simulink model "SNL_S_Function"  (R2020b)
settings: Solver=VariableStepAuto  StartTime=0.0  StopTime=10.0  RelTol=1e-3
settings Model: Creator=ashahn  LastModifiedBy=ashahn

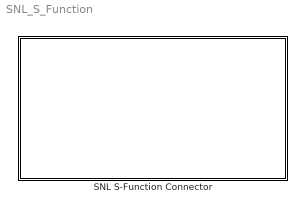
== system SNL_S_Function ==
  SNL S-Function Connector : Subsystem

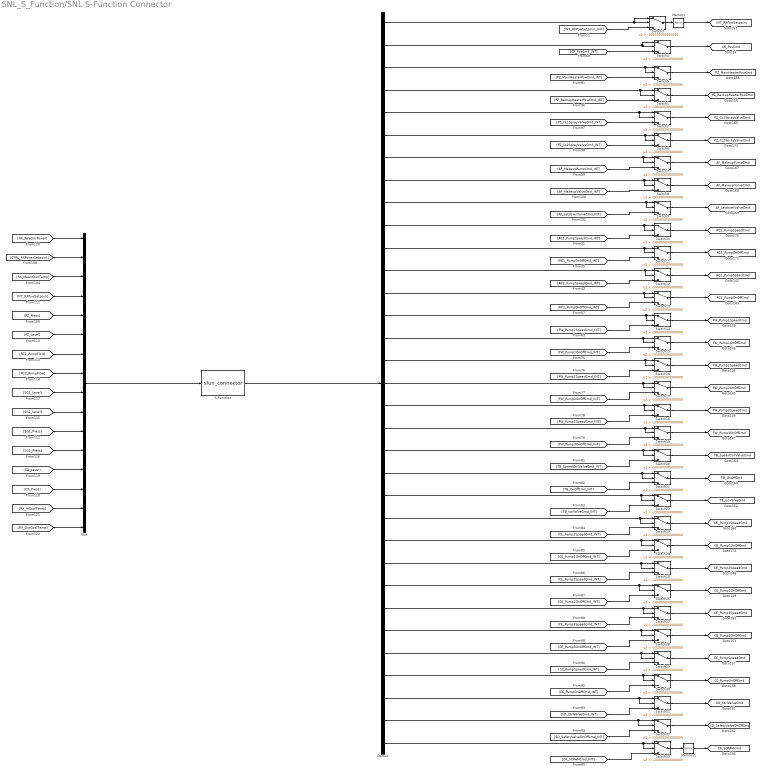
== system SNL_S_Function/SNL S-Function Connector ==
  Demux : Demux  Outputs=33
  Memory : Memory
  Memory1 : Memory
  Mux : Mux  Inputs=16
  S-Function : S-Function  FunctionName=sfun_connector  Parameters='RX_ReactorPower;CTRL_RXPowerSetpoint;RX_MeanCoolTemp;INT_RXPowSetpoint;PZ_Press;PZ_Level;RC1_PumpFlow;RC2_PumpFlow;SG1_Level;SG2_Level;SG1_Press;SG2_Press;CD_Level;CD_Press;RX_InCoolTemp;RX_OutCoolTemp','INT_RXPowSetpoint;CR_PosCmd;PZ_MainHeaterPowCmd;PZ_BackupHeaterPowCmd;PZ_CL1SprayValveCmd;PZ_CL2SprayValveCmd;AF_MakeupPumpCmd;AF_MakeupValveCmd;AF_LetdownValveCmd;RC1_PumpSpeedCmd;RC1_PumpOnOffCmd;RC2_PumpSpeedCmd;RC2_PumpOnOffCmd;FW_Pump1SpeedCmd;FW_Pump1OnOffCmd;FW_Pump2SpeedCmd;FW_Pump2OnOffCmd;FW_Pump3SpeedCmd;FW_Pump3OnOffCmd;TB_SpeedCtrlValveCmd;TB_OnOffCmd;TB_IsoValveCmd;CE_Pump1SpeedCmd;CE_Pump1OnOffCmd;CE_Pump2SpeedCmd;CE_Pump2OnOffCmd;CE_Pump3SpeedCmd;CE_Pump3OnOffCmd;CC_PumpSpeedCmd;CC_PumpOnOffCmd;SD_CtrlValveCmd;SD_SafetyValveOnOffCmd;CR_SCRAMCmd'  SFunctionDeploymentMode=off  EnableBusSupport=off
  Switch{1..33} (33 alike) : Switch  Criteria=u2 > Threshold  Threshold=-100000000000000
  tag scope: AF_LetdownValveCmd=global, AF_MakeupPumpCmd=global, AF_MakeupValveCmd=global, CC_PumpOnOffCmd=global, CC_PumpSpeedCmd=global, CE_Pump1OnOffCmd=global, CE_Pump1SpeedCmd=global, CE_Pump2OnOffCmd=global, CE_Pump2SpeedCmd=global, CE_Pump3OnOffCmd=global, CE_Pump3SpeedCmd=global, CR_PosCmd=global, CR_SCRAMCmd=global, FW_Pump1OnOffCmd=global, FW_Pump1SpeedCmd=global, FW_Pump2OnOffCmd=global, FW_Pump2SpeedCmd=global, FW_Pump3OnOffCmd=global, FW_Pump3SpeedCmd=global, INT_RXPowSetpoint=global, PZ_BackupHeaterPowCmd=global, PZ_CL1SprayValveCmd=global, PZ_CL2SprayValveCmd=global, PZ_MainHeaterPowCmd=global, RC1_PumpOnOffCmd=global, RC1_PumpSpeedCmd=global, RC2_PumpOnOffCmd=global, RC2_PumpSpeedCmd=global, SD_CtrlValveCmd=global, SD_SafetyValveOnOffCmd=global, TB_IsoValveCmd=global, TB_OnOffCmd=global, TB_SpeedCtrlValveCmd=global
  wires:
  [PZ_Level] -> Mux/6
  Demux/29 -> Switch29/2, Switch29/1
  Switch24/1 -> [CE_Pump1OnOffCmd]
  [PZ_CL1SprayValveCmd_INT] -> Switch2/3
  Switch13/1 -> [RC2_PumpOnOffCmd]
  Switch28/1 -> [CE_Pump3OnOffCmd]
  Switch19/1 -> [FW_Pump3OnOffCmd]
  Demux/6 -> Switch6/2, Switch6/1
  Switch12/1 -> [RC2_PumpSpeedCmd]
  [FW_Pump2OnOffCmd_INT] -> Switch17/3
  Demux/22 -> Switch22/2, Switch22/1
  Demux/13 -> Switch13/2, Switch13/1
  [FW_Pump1OnOffCmd_INT] -> Switch15/3
  Demux/30 -> Switch30/2, Switch30/1
  [RX_ReactorPower] -> Mux/1
  Demux/8 -> Switch8/2, Switch8/1
  Switch29/1 -> [CC_PumpSpeedCmd]
  [CE_Pump1SpeedCmd_INT] -> Switch23/3
  Switch14/1 -> [FW_Pump1SpeedCmd]
  Switch26/1 -> [CE_Pump2OnOffCmd]
  [TB_SpeedCtrlValveCmd_INT] -> Switch20/3
  [RX_MeanCoolTemp] -> Mux/3
  Demux/32 -> Switch32/2, Switch32/1
  [CC_PumpOnOffCmd_INT] -> Switch30/3
  Switch1/1 -> [PZ_BackupHeaterPowCmd]
  [CTRL_RXPowerSetpoint] -> Mux/2
  [SG2_Level] -> Mux/10
  [CE_Pump3SpeedCmd_INT] -> Switch27/3
  [SG1_Level] -> Mux/9
  Demux/16 -> Switch16/2, Switch16/1
  Switch6/1 -> [PZ_CL2SprayValveCmd]
  Switch17/1 -> [FW_Pump2OnOffCmd]
  [CE_Pump1OnOffCmd_INT] -> Switch24/3
  [FW_Pump3OnOffCmd_INT] -> Switch19/3
  [PZ_MainHeaterPowCmd_INT] -> Switch5/3
  Switch16/1 -> [FW_Pump2SpeedCmd]
  [FW_Pump2SpeedCmd_INT] -> Switch16/3
  [CE_Pump3OnOffCmd_INT] -> Switch28/3
  Switch25/1 -> [CE_Pump2SpeedCmd]
  Switch7/1 -> [AF_MakeupPumpCmd]
  Demux/19 -> Switch19/2, Switch19/1
  Demux/15 -> Switch15/2, Switch15/1
  [SD_SafetyValveOnOffCmd_INT] -> Switch32/3
  [CE_Pump2SpeedCmd_INT] -> Switch25/3
  Demux/12 -> Switch12/2, Switch12/1
  Demux/17 -> Switch17/2, Switch17/1
  Switch9/1 -> [AF_LetdownValveCmd]
  Switch22/1 -> [TB_IsoValveCmd]
  Switch30/1 -> [CC_PumpOnOffCmd]
  [RX_OutCoolTemp] -> Mux/16
  Demux/25 -> Switch25/2, Switch25/1
  Switch4/1 -> [CR_PosCmd]
  [AF_LetdownValveCmd_INT] -> Switch9/3
  [RC1_PumpSpeedCmd_INT] -> Switch10/3
  [RC2_PumpSpeedCmd_INT] -> Switch12/3
  Demux/3 -> Switch5/2, Switch5/1
  Demux/31 -> Switch31/2, Switch31/1
  [RC2_PumpOnOffCmd_INT] -> Switch13/3
  [TB_IsoValveCmd_INT] -> Switch22/3
  Demux/9 -> Switch9/2, Switch9/1
  [CD_Level] -> Mux/13
  [TB_OnOffCmd_INT] -> Switch21/3
  Switch2/1 -> [PZ_CL1SprayValveCmd]
  Demux/4 -> Switch1/2, Switch1/1
  Demux/26 -> Switch26/2, Switch26/1
  Switch15/1 -> [FW_Pump1OnOffCmd]
  [CC_PumpSpeedCmd_INT] -> Switch29/3
  Switch8/1 -> [AF_MakeupValveCmd]
  Switch23/1 -> [CE_Pump1SpeedCmd]
  [CD_Press] -> Mux/14
  Switch20/1 -> [TB_SpeedCtrlValveCmd]
  Switch10/1 -> [RC1_PumpSpeedCmd]
  Demux/2 -> Switch4/1, Switch4/2
  Demux/28 -> Switch28/2, Switch28/1
  [FW_Pump1SpeedCmd_INT] -> Switch14/3
  Switch31/1 -> [SD_CtrlValveCmd]
  Mux/1 -> S-Function/1
  Switch21/1 -> [TB_OnOffCmd]
  [SG2_Press] -> Mux/12
  [RC2_PumpFlow] -> Mux/8
  [SD_CtrlValveCmd_INT] -> Switch31/3
  Demux/5 -> Switch2/2, Switch2/1
  Demux/21 -> Switch21/2, Switch21/1
  Demux/27 -> Switch27/2, Switch27/1
  [AF_MakeupValveCmd_INT] -> Switch8/3
  Switch11/1 -> [RC1_PumpOnOffCmd]
  Demux/10 -> Switch10/2, Switch10/1
  [FW_Pump3SpeedCmd_INT] -> Switch18/3
  Switch27/1 -> [CE_Pump3SpeedCmd]
  [RC1_PumpFlow] -> Mux/7
  Demux/1 -> Switch3/1, Switch3/2
  [CE_Pump2OnOffCmd_INT] -> Switch26/3
  [RC1_PumpOnOffCmd_INT] -> Switch11/3
  S-Function/1 -> Demux/1
  Switch32/1 -> [SD_SafetyValveOnOffCmd]
  Demux/20 -> Switch20/2, Switch20/1
  Demux/7 -> Switch7/2, Switch7/1
  [SG1_Press] -> Mux/11
  Demux/18 -> Switch18/2, Switch18/1
  Demux/23 -> Switch23/2, Switch23/1
  [RX_InCoolTemp] -> Mux/15
  [PZ_Press] -> Mux/5
  Switch5/1 -> [PZ_MainHeaterPowCmd]
  [PZ_BackupHeaterPowCmd_INT] -> Switch1/3
  Demux/14 -> Switch14/2, Switch14/1
  Switch18/1 -> [FW_Pump3SpeedCmd]
  [AF_MakeupPumpCmd_INT] -> Switch7/3
  Demux/24 -> Switch24/2, Switch24/1
  [PZ_CL2SprayValveCmd_INT] -> Switch6/3
  Demux/11 -> Switch11/2, Switch11/1
  [INT_RXPowSetpoint] -> Mux/4
  [CR_PosCmd_INT] -> Switch4/3
  Switch3/1 -> Memory/1
  Demux/33 -> Switch33/2, Switch33/1
  Switch33/1 -> Memory1/1
  Memory/1 -> [INT_RXPowSetpoint]
  [INT_RXPowSetpoint_INT] -> Switch3/3
  Memory1/1 -> [CR_SCRAMCmd]
  [CR_SCRAMCmd_INT] -> Switch33/3
